simulink model "lab1"  (R2022a)
settings: Solver=VariableStepAuto  StartTime=0.0  StopTime=Tmdl  MaxStep=0.001  RelTol=1e-3
undefined symbols (not defined in the file): J1, J2, k12
libraries: slctrlblks x1
settings Model: Creator=81502  LastModifiedBy=81502

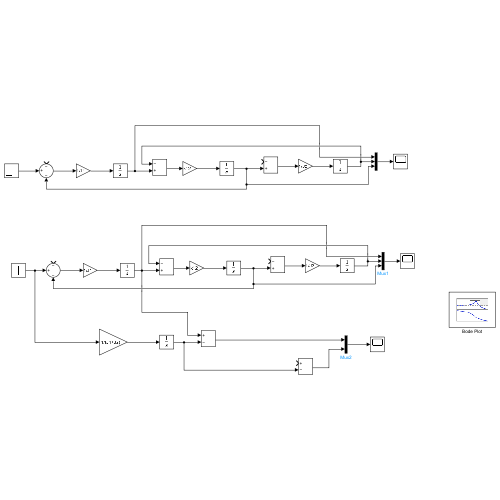
[thumbnail: Simulink's stored preview of the top-level diagram]
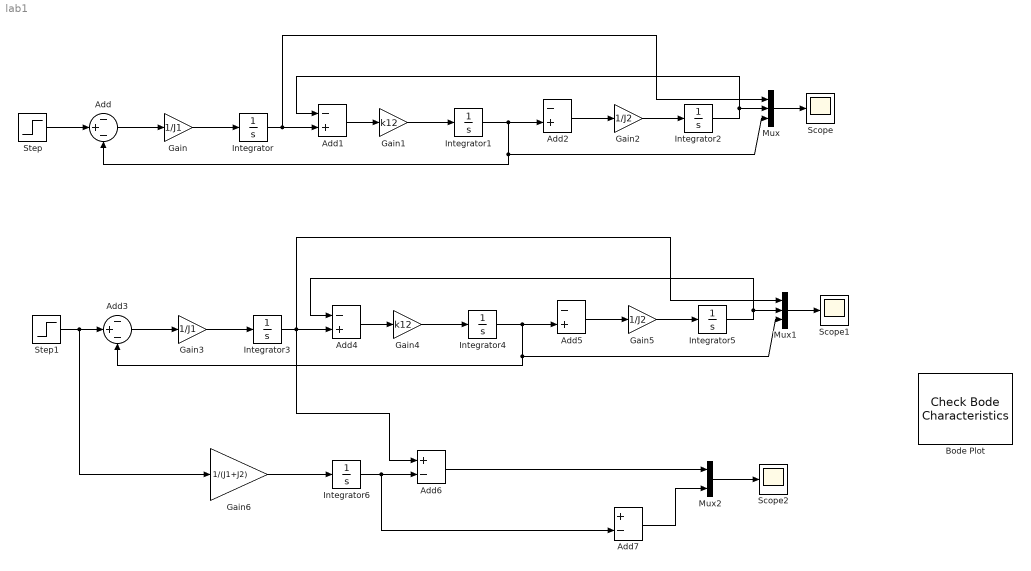
== system lab1 ==
  Add : Sum  Inputs=-+-
  Add{1..2,4..5} (4 alike) : Sum  Inputs=-+
  Add3 : Sum  Inputs=-+-
  Add6 : Sum  Inputs=+-
  Add7 : Sum  Inputs=+-
  Bode Plot : slctrlblks/Model Verification/Check Bode  Characteristics  InstantiateOnLoad=on  SaveOperatingPoints=off  LinearizationIOs={}  LinearizeAt=SnapshotTimes  SnapshotTimes=[0]  TriggerType=rising  SampleTime=auto  RateConversionMethod=zoh  PreWarpFreq=10  UseExactDelayModel=off  UseFullBlockNameLabels=off  UseBusSignalLabels=off  enabled=on  stopWhenAssertionFail=off  export=off  ViewDlgPos=[193.8 205.8 509.6 389.6]  OpenViewOnLoad=off  LaunchViewOnOpen=on  FrequencyUnits=rad/s  MagnitudeUnits=dB  PhaseUnits=deg  TimeUnits=seconds  EnableUpperBound=off  UpperBoundFrequencies=[]  UpperBoundMagnitudes=[]  EnableLowerBound=off  LowerBoundFrequencies=[]  LowerBoundMagnitudes=[]
  Gain : Gain  Gain=1/J1
  Gain1 : Gain  Gain=k12
  Gain2 : Gain  Gain=1/J2
  Gain3 : Gain  Gain=1/J1
  Gain4 : Gain  Gain=k12
  Gain5 : Gain  Gain=1/J2
  Gain6 : Gain  Gain=1/(J1+J2)
  Integrator{,1..6} (7 alike) : Integrator
  Mux : Mux  Inputs=3
  Mux1 : Mux  Inputs=3
  Mux2 : Mux  Inputs=2
  Scope : Scope
  Scope1 : Scope
  Scope2 : Scope
  Step : Step  SampleTime=0
  Step1 : Step  SampleTime=0
  wires:
  Gain/1 -> Integrator/1
  Add/1 -> Gain/1
  Step/1 -> Add/2
  Add1/1 -> Gain1/1
  Gain1/1 -> Integrator1/1
  Integrator1/1 -> Add/3, Mux/3, Add2/2
  Add2/1 -> Gain2/1
  Gain2/1 -> Integrator2/1
  Integrator2/1 -> Add1/1, Mux/2
  Integrator/1 -> Mux/1, Add1/2
  Mux/1 -> Scope/1
  Integrator5/1 -> Add4/1, Mux1/2
  Gain3/1 -> Integrator3/1
  Step1/1 -> Gain6/1, Add3/2
  Add4/1 -> Gain4/1
  Integrator4/1 -> Add3/3, Mux1/3, Add5/2
  Mux1/1 -> Scope1/1
  Gain4/1 -> Integrator4/1
  Add5/1 -> Gain5/1
  Integrator3/1 -> Add6/1, Mux1/1, Add4/2
  Gain5/1 -> Integrator5/1
  Add3/1 -> Gain3/1
  Gain6/1 -> Integrator6/1
  Integrator6/1 -> Add7/2, Add6/2
  Add6/1 -> Mux2/1
  Add7/1 -> Mux2/2
  Mux2/1 -> Scope2/1
